simulink model "simulateur"  (R2023a)
settings: Solver=ode45  StartTime=0.0  StopTime=10  RelTol=1e-5  AbsTol=1e-5  EnableMultiTasking=on
values from neighbouring files (symbols this model uses):
  control = [control.Time control.Data]    [anim.m]    (also in control.m = inv(B)*(-qs*qv+cross(w,J*w)+J*Kq*dqv-K*(w-Kq*qv)))
settings Model: Creator=pmorin  LastModifiedBy=haoyuan
settings SolverCC: AlgebraicLoopSolver=TrustRegion
settings DataIOCC: LimitDataPoints=on  SaveFormat=Array  SignalLoggingSaveFormat=ModelDataLogs  ReturnWorkspaceOutputs=off
settings OptimizationCC: BooleanDataType=off
settings DebuggingCC: SaveWithParameterizedLinksMsg=none  UnderspecifiedInitializationDetection=Classic  MergeDetectMultiDrivingBlocksExec=none  SignalResolutionControl=TryResolveAllWithWarning  MultiTaskDSMMsg=warning  MultiTaskCondExecSysMsg=none  UnconnectedInputMsg=warning  UnconnectedOutputMsg=warning  UnconnectedLineMsg=warning
settings HardwareCC: TargetUnknown=on
settings ModelReferenceCC: EnableRefExpFcnMdlSchedulingChecks=on  PropagateSignalLabelsOutOfModel=off
settings GRTTargetCC: CombineOutputUpdateFcns=off  GRTInterface=on
settings ConfigComp: CovMetricSettings=dw

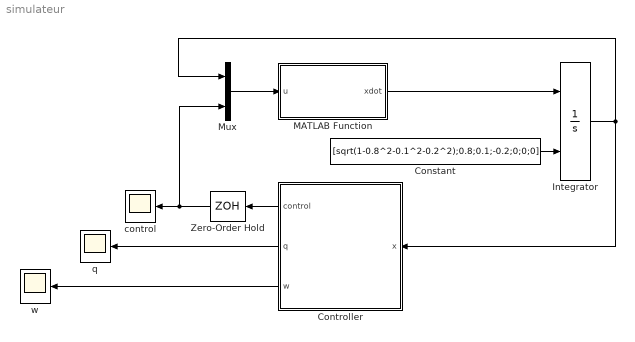
== system simulateur ==
  Constant : Constant  Value=[sqrt(1-0.8^2-0.1^2-0.2^2);0.8;0.1;-0.2;0;0;0]
  Controller : Subsystem
  Integrator : Integrator  InitialConditionSource=external
  MATLAB Function : MATLAB Function  TreatAsAtomicUnit=on
  Mux : Mux  Inputs=2
  Zero-Order Hold : ZeroOrderHold  SampleTime=0.1
  control : Scope
  q : Scope
  w : Scope
  wires:
  Controller/2(q) -> q/1
  Mux/1 -> MATLAB Function/1(u)
  MATLAB Function/1(xdot) -> Integrator/1
  Constant/1 -> Integrator/2
  Controller/3(w) -> w/1
  Controller/1(control) -> Zero-Order Hold/1
  Integrator/1 -> Controller/1(x), Mux/1
  Zero-Order Hold/1 -> Mux/2, control/1

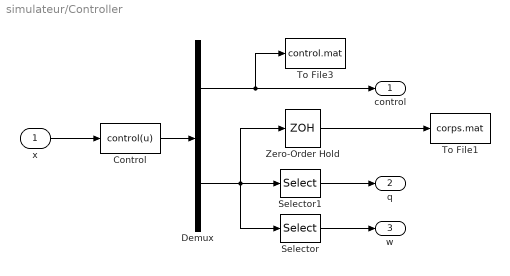
== system simulateur/Controller ==
  x : Inport
  Control : MATLABFcn  MATLABFcn=control(u)  OutputDimensions=10
  Demux : Demux  Outputs=[3 7]
      settings: DisplayOption=none
  Selector : Selector  InputPortWidth=7  IndexOptions=Index vector (dialog)  Indices=[5 6 7]  OutputSizes=1
  Selector1 : Selector  InputPortWidth=7  IndexOptions=Index vector (dialog)  Indices=[1 2 3 4]  OutputSizes=1
  To File1 : ToFile  Filename=corps.mat  SaveFormat=Timeseries
  To File3 : ToFile  Filename=control.mat  SaveFormat=Timeseries
  Zero-Order Hold : ZeroOrderHold  SampleTime=0.01
  control : Outport
  q : Outport  Port=2
  w : Outport  Port=3
  wires:
  Zero-Order Hold/1 -> To File1/1
  Demux/2 -> Selector/1, Zero-Order Hold/1, Selector1/1
  Control/1 -> Demux/1
  Demux/1 -> To File3/1, control/1
  Selector/1 -> w/1
  x/1 -> Control/1
  Selector1/1 -> q/1

== matlab function simulateur/MATLAB Function ==
  data: u input; xdot output
function xdot= dynamique(u)
% Fonction qui définit la dynamique du corps à contrôler

% On définit les paramètres mécaniques du corps
J= [1 -1 0; -1 2 1; 0 1 2];
B= [1 0 0.2;0.1 1 0; -0.1 -0.2 1];

% On redéfinit les états en fonction de u:
qs= u(1);
qv= u(2:4);
w= u(5:7);
control= u(8:10);

% On définit la dynamique du corps avec un terme de correction
dqs= -0.5*qv'*w-qs*(norm([qs;qv])^2-1);
dqv= 0.5*(qs*w+cross(qv,w))-qv*(norm([qs;qv])^2-1);
dw= inv(J)*(-cross(w, J*w)+B*control);

xdot = [dqs;dqv;dw];
